simulink subsystem "outerLoop"  (R2026a)
settings: Solver=VariableStepAuto
settings Model: Creator=maxhu  LastModifiedBy=maxhu

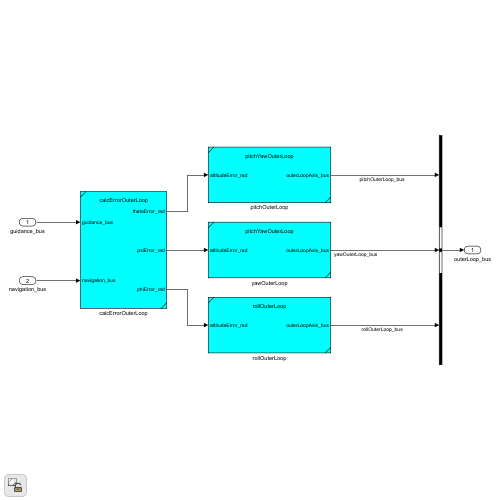
[thumbnail: Simulink's stored preview of the top-level diagram]
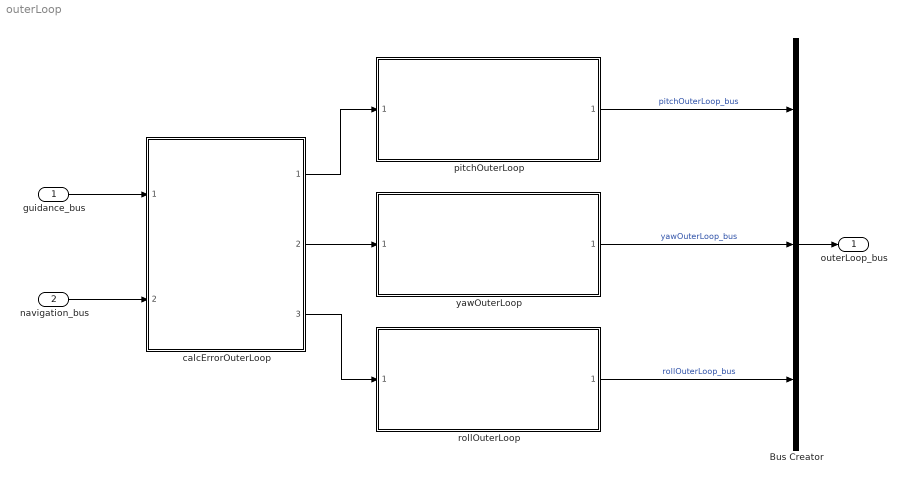
== system outerLoop ==
  guidance_bus : Inport
  navigation_bus : Inport  Port=2
  Bus Creator : BusCreator  Inputs=3
  calcErrorOuterLoop : Subsystem  ReferencedSubsystem=calcErrorOuterLoop
  pitchOuterLoop : Subsystem  ReferencedSubsystem=pitchYawOuterLoop
      settings: PermitHierarchicalResolution=None
  rollOuterLoop : Subsystem  ReferencedSubsystem=rollOuterLoop
      settings: PermitHierarchicalResolution=None
  yawOuterLoop : Subsystem  ReferencedSubsystem=pitchYawOuterLoop
      settings: PermitHierarchicalResolution=None
  outerLoop_bus : Outport
  wires:
  pitchOuterLoop/1 -> Bus Creator/1  "pitchOuterLoop_bus"
  rollOuterLoop/1 -> Bus Creator/3  "rollOuterLoop_bus"
  Bus Creator/1 -> outerLoop_bus/1
  guidance_bus/1 -> calcErrorOuterLoop/1
  navigation_bus/1 -> calcErrorOuterLoop/2
  calcErrorOuterLoop/3 -> rollOuterLoop/1
  calcErrorOuterLoop/1 -> pitchOuterLoop/1
  yawOuterLoop/1 -> Bus Creator/2  "yawOuterLoop_bus"
  calcErrorOuterLoop/2 -> yawOuterLoop/1
